simulink model "rSteeringAngle"  (R2024b)
settings: configuration reference "STM32H7_Config" (kept outside this file)
undefined symbols (not defined in the file): aSteeringAngleMax, rSteeringAngleCalHigh, rSteeringAngleCalLow, VSteeringAngleHighSample, VSteeringAngleLowSample
settings Model: DataDictionary=Master_Dictionary.sldd  EnableAccessToBaseWorkspace=off  Creator=torni  LastModifiedBy=William
settings ConfigSetRef: SourceName=STM32H7_Config

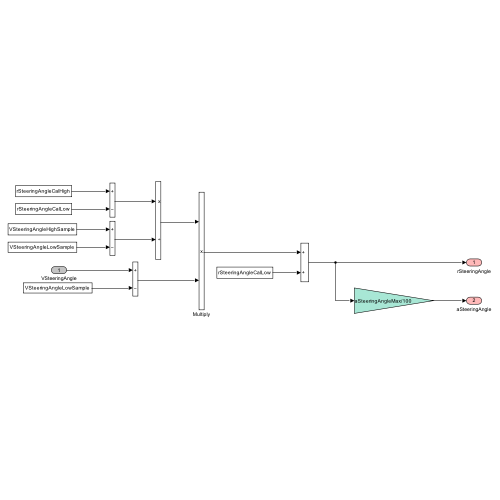
[thumbnail: Simulink's stored preview of the top-level diagram]
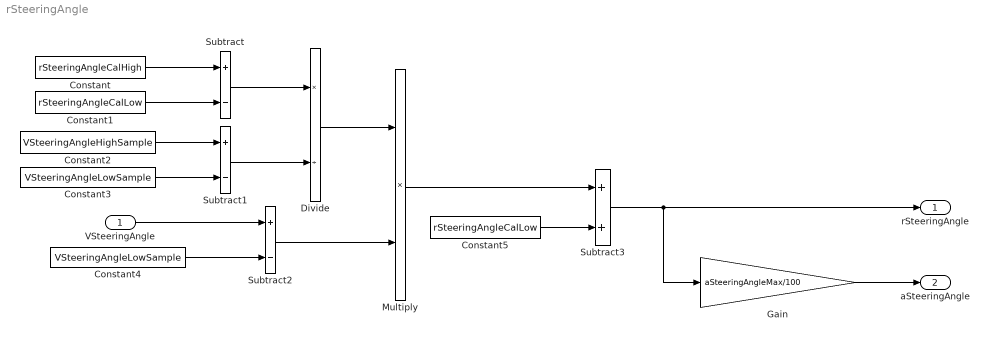
== system rSteeringAngle ==
  VSteeringAngle : Inport  OutDataTypeStr=double
  Constant : Constant  Value=rSteeringAngleCalHigh
  Constant1 : Constant  Value=rSteeringAngleCalLow
  Constant2 : Constant  Value=VSteeringAngleHighSample
  Constant3 : Constant  Value=VSteeringAngleLowSample
  Constant4 : Constant  Value=VSteeringAngleLowSample
  Constant5 : Constant  Value=rSteeringAngleCalLow
  Divide : Product  Inputs=*/
  Gain : Gain  Gain=aSteeringAngleMax/100
  Multiply : Product
  Subtract : Sum  Inputs=+-
  Subtract1 : Sum  Inputs=+-
  Subtract2 : Sum  Inputs=+-
  Subtract3 : Sum
  rSteeringAngle : Outport  OutDataTypeStr=double  VectorParamsAs1DForOutWhenUnconnected=off
  aSteeringAngle : Outport  Port=2  OutDataTypeStr=double  VectorParamsAs1DForOutWhenUnconnected=off
  wires:
  Gain/1 -> aSteeringAngle/1
  Constant3/1 -> Subtract1/2
  Divide/1 -> Multiply/1
  Subtract1/1 -> Divide/2
  Constant4/1 -> Subtract2/2
  Multiply/1 -> Subtract3/1
  Subtract/1 -> Divide/1
  Constant2/1 -> Subtract1/1
  Constant/1 -> Subtract/1
  Constant5/1 -> Subtract3/2
  Subtract2/1 -> Multiply/2
  Constant1/1 -> Subtract/2
  VSteeringAngle/1 -> Subtract2/1
  Subtract3/1 -> Gain/1, rSteeringAngle/1
